simulink model "WallTimeDemo"  (Simulink 7.3)
settings: Solver=FixedStepDiscrete  StartTime=0.0  StopTime=inf  FixedStep=0.005  RelTol=1e-3
undefined symbols (not defined in the file or in its folder): datevec
libraries: xpcwalltimelib x4, xpclib x2
settings Model: Creator=jraichek  LastModifiedBy=jraichek  BufferReuse=off
settings OptimizationCC: BlockReduction=off  OptimizeBlockIOStorage=off  BufferReuse=off  ExpressionFolding=off  LocalBlockOutputs=off
settings HardwareCC: ProdIntDivRoundTo=Zero  ProdEndianess=LittleEndian  ProdHWDeviceType=Generic->32-bit x86 compatible
settings RTWCC: SystemTargetFile=xpctarget.tlc  TemplateMakefile=xpc_default_tmf  Description=xPC Target  ProcessScript=xpctarget_make_rtw_hook  RTWCompilerOptimization=On
settings xpcTargetCC: TargetFcnLib=ansi_tfl_table_tmw.mat  TargetFunctionLibrary=ANSI_C  PortableWordSizes=off

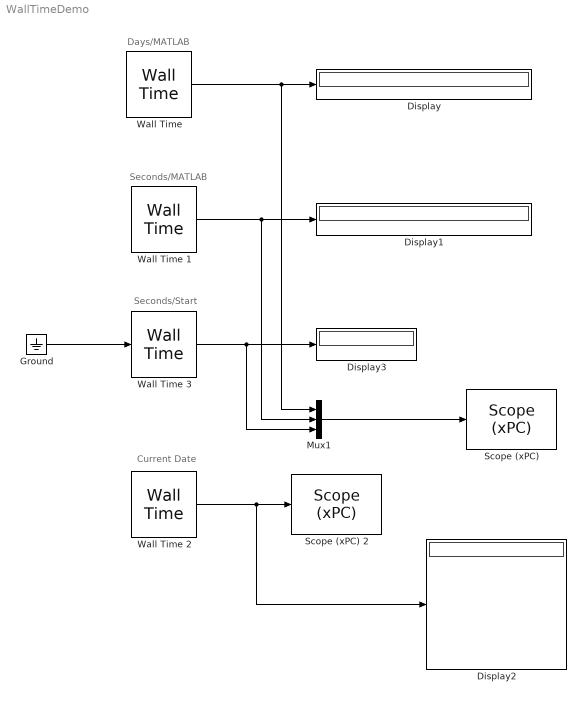
== system WallTimeDemo ==
  note: Days/MATLAB
  note: Seconds/MATLAB
  note: Current Date
  note: Seconds/Start
  Display{,1..3} (4 alike) : Display
      Display settings: Format=long_e
      Display1 settings: Format=long_e
  Ground : Ground
  Mux1 : Mux  Inputs=3
  "Scope (xPC) " : xpclib/Misc./Scope (xPC)   SystemSampleTime=-1  scopeno=1  scopetype=Target  autostart=on  viewmode=Numerical  formatstr="' Days since Epoch:       %15.6f, Seconds since Epoch: %15.6f, Seconds since Block Start: %6.6f'"  grid=on  ylimits=[0,0]  nosamples=10  noprepostsamples=0  interleave=1  triggermode=FreeRun  triggersignal=1  triggerlevel=0.0  triggerslope=Either  triggerscope=1  triggersample=0  filename=data.dat  mode=Lazy  writesize=512  autorestart=off
  Scope (xPC) 2 : xpclib/Misc./Scope (xPC)   SystemSampleTime=-1  scopeno=3  scopetype=Target  autostart=on  viewmode=Numerical  formatstr="' Current Year: %4.0f, Current Month:  %2.0f, Current Day:    %2.0f, Current Hour:   %2.0f, Current Min:    %2.0f, Current Sec:    %2.0f'"  grid=on  ylimits=[0,0]  nosamples=10  noprepostsamples=0  interleave=1  triggermode=FreeRun  triggersignal=1  triggerlevel=0.0  triggerslope=Either  triggerscope=1  triggersample=0  filename=data.dat  mode=Lazy  writesize=512  autorestart=off
  "Wall Time " : xpcwalltimelib/Wall Time   TimeFormat=Days  EpochSource=MATLAB  EpochVector=datevec('01/01/1970')  InputTrigger=off  SampleTime=0.005
  Wall Time 1 : xpcwalltimelib/Wall Time   TimeFormat=Seconds  EpochSource=MATLAB  EpochVector=datevec('01/01/1970')  InputTrigger=off  SampleTime=0.005
  Wall Time 2 : xpcwalltimelib/Wall Time   TimeFormat=Date  EpochSource=MATLAB  EpochVector=datevec('01/01/1970')  InputTrigger=off  SampleTime=0.005
  Wall Time 3 : xpcwalltimelib/Wall Time   TimeFormat=Seconds  EpochSource=Start  EpochVector=datevec('01/01/1970')  InputTrigger=on  SampleTime=0.001
  wires:
  Wall Time 2/1 -> Scope (xPC) 2/1, Display2/1
  Ground/1 -> Wall Time 3/1
  "Wall Time "/1 -> Display/1, Mux1/1
  Wall Time 1/1 -> Display1/1, Mux1/2
  Wall Time 3/1 -> Display3/1, Mux1/3
  Mux1/1 -> "Scope (xPC) "/1
